simulink model "wristposition"  (R2023a)
settings: Solver=VariableStepAuto  StartTime=0.0  StopTime=1  RelTol=1e-3
undefined symbols (not defined in the file): x_in
settings Model: Creator=s202421  LastModifiedBy=s202421

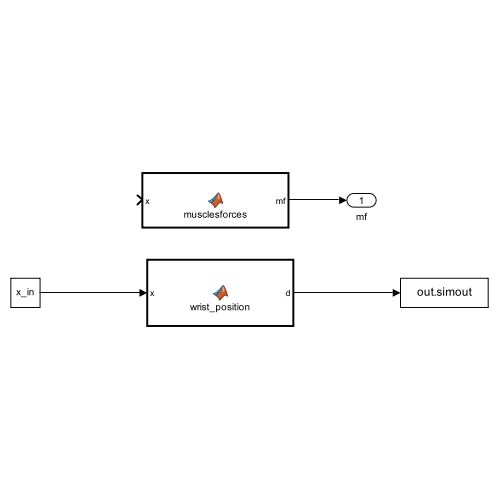
[thumbnail: Simulink's stored preview of the top-level diagram]
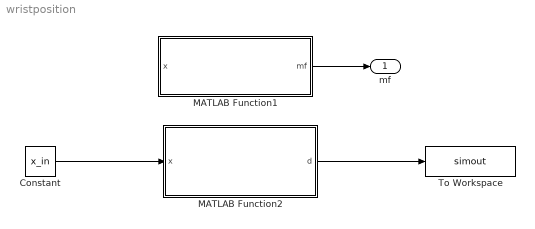
== system wristposition ==
  Constant : Constant  Value=x_in
  MATLAB Function1 : MATLAB Function  TreatAsAtomicUnit=on
  MATLAB Function2 : MATLAB Function  TreatAsAtomicUnit=on
  To Workspace : ToWorkspace  VariableName=simout  SaveFormat=Timeseries  SampleTime=-1
  mf : Outport
  wires:
  Constant/1 -> MATLAB Function2/1(x)
  MATLAB Function2/1(d) -> To Workspace/1
  MATLAB Function1/1(mf) -> mf/1

== matlab function wristposition/MATLAB Function2 ==
  data: d output; x input
function d = wrist_position(x)
    coder.extrinsic('das3')
    d = zeros(13,12);
    d = das3('Visualization',x);
    j = length(d);

    p = d(j,1:3)';					% position vector of bone
	R = reshape(d(j,4:12),3,3)';	% orientation matrix
	
	create n x 3 matrix of the bone points local coordinates
	plocal =  [0,0,0; 0.0171, -0.0133, -0.0163]';
	npoints =  2;
	
	transform to global coordinates
	pglobal = repmat(p,1,npoints) + R*plocal;
    x = pglobal(3,2);
    y = pglobal(1,2);
    z = pglobal(2,2);
    pos = x;

== matlab function wristposition/MATLAB Function1 ==
  data: x input; mf output
function mf = musclesforces(x)
    mf = das3('Muscleforces',x);
